simulink subsystem "WindTurbine"  (R2023b)
settings: Solver=VariableStepAuto  StartTime=0.0  StopTime=10.0  RelTol=1e-3
values from neighbouring files (symbols this model uses):
  brakePressure = 100    [wind_turbine_inputs.m]
  generatorEfficiency = 90    [wind_turbine_inputs.m]
  generatorLumpedInductance = 1.9160e-04    (= 0.0001916)    [wind_turbine_inputs.m]
  generatorLumpedResistance = 0.0027    [wind_turbine_inputs.m]
  gridFrequency = 60    [wind_turbine_inputs.m]
  turbineRadius = 70.5/2    (= 35.25)    [wind_turbine_inputs.m]
  turbineRatedPower = 1.5    [wind_turbine_inputs.m]
  wAtGeneratorRatedPower = wTurbineCutOut*gearRatio    (= 1227.93)    [wind_turbine_inputs.m]
undefined symbols (not defined in the file or in its folder): ee_sli_rtmsupport, G, gcbh, X, Y, Z
libraries: sm_lib x42, fl_lib x17, nesl_utility x10, sdl_lib x6, ee_lib x6, simulink x4, eeGeneralControl x3, eeGeneralMeasurement x2
(part 2 of 2)

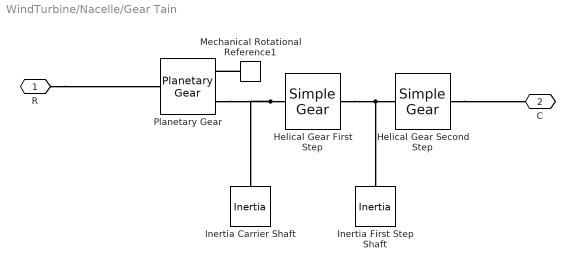
== system WindTurbine/Nacelle/Gear Tain ==
  Helical Gear First Step : sdl_lib/Gears/Simple Gear  ratio=firstStepTeethRatio  rotation_direction=sdl.enum.shaftOutputDirection.opposite  friction_model=sdl.enum.gear_efficiencies_load.constant  T_noload=0.1 N*m  T_nom=5 N*m  efficiency_nom=0.8  efficiency=0.95  temperature_TLU=[ 280 300 320 ] K  load_TLU=[ 1 5 10 ] N*m  efficiency_TLU=[ 0.95 0.9 0.85 ]  efficiency_TLU2=[ 0.85 0.8 0.75; 0.95 0.9 0.85; 0.85 0.8 0.7 ]  w_thr=0.01 rad/s  pwr_thr=0.001 W  enable_backlash=false  hardstop_model=simscape.enum.hardstop.smooth  backlash_distance=1e-3 mm  r_base=0.1 m  transition=1e-4 mm  backlash_stiffness=1e7 N/m  backlash_damping=1e6 N/(m/s)  coeff_rest=0  v_tol=0.001 m/s  f_tol=0 N  mu_visc=[ 0 0 ] N*m/(rad/s)  enable_faults=simscape.enum.onoff.off  efficiency_fault=0.05  external_fault=simscape.enum.onoff.off  temporal_fault=simscape.enum.onoff.off  fault_time=5 s  fault_angles=pi / 12 rad  report_fault=simscape.enum.assert.action.none  thermal_mass=50 J/K  temperature_specify=off  temperature_priority=High  temperature=300 K  temperature_nominal_specify=off  temperature_nominal_unit=K  temperature_nominal_value=1  x_backlash_specify=off  x_backlash_priority=None  x_backlash=0 mm  x_backlash_nominal_specify=off  x_backlash_nominal_unit=mm  x_backlash_nominal_value=1  f_hardstop_specify=off  f_hardstop_priority=None  f_hardstop=0 N  f_hardstop_nominal_specify=off  f_hardstop_nominal_unit=N  f_hardstop_nominal_value=1  v_backlash_specify=off  v_backlash_priority=None  v_backlash=0 m/s  v_backlash_nominal_specify=off  v_backlash_nominal_unit=m/s  v_backlash_nominal_value=1
  Helical Gear Second Step : sdl_lib/Gears/Simple Gear  ratio=secondStepTeethRatio  rotation_direction=sdl.enum.shaftOutputDirection.same  friction_model=sdl.enum.gear_efficiencies_load.constant  T_noload=0.1 N*m  T_nom=5 N*m  efficiency_nom=0.8  efficiency=0.95  temperature_TLU=[ 280 300 320 ] K  load_TLU=[ 1 5 10 ] N*m  efficiency_TLU=[ 0.95 0.9 0.85 ]  efficiency_TLU2=[ 0.85 0.8 0.75; 0.95 0.9 0.85; 0.85 0.8 0.7 ]  w_thr=0.01 rad/s  pwr_thr=0.001 W  enable_backlash=false  hardstop_model=simscape.enum.hardstop.smooth  backlash_distance=1e-3 mm  r_base=0.1 m  transition=1e-4 mm  backlash_stiffness=1e7 N/m  backlash_damping=1e6 N/(m/s)  coeff_rest=0  v_tol=0.001 m/s  f_tol=0 N  mu_visc=[ 0 0 ] N*m/(rad/s)  enable_faults=simscape.enum.onoff.off  efficiency_fault=0.05  external_fault=simscape.enum.onoff.off  temporal_fault=simscape.enum.onoff.off  fault_time=5 s  fault_angles=pi / 12 rad  report_fault=simscape.enum.assert.action.none  thermal_mass=50 J/K  temperature_specify=off  temperature_priority=High  temperature=300 K  temperature_nominal_specify=off  temperature_nominal_unit=K  temperature_nominal_value=1  x_backlash_specify=off  x_backlash_priority=None  x_backlash=0 mm  x_backlash_nominal_specify=off  x_backlash_nominal_unit=mm  x_backlash_nominal_value=1  f_hardstop_specify=off  f_hardstop_priority=None  f_hardstop=0 N  f_hardstop_nominal_specify=off  f_hardstop_nominal_unit=N  f_hardstop_nominal_value=1  v_backlash_specify=off  v_backlash_priority=None  v_backlash=0 m/s  v_backlash_nominal_specify=off  v_backlash_nominal_unit=m/s  v_backlash_nominal_value=1
  Inertia Carrier Shaft : fl_lib/Mechanical/Rotational Elements/Inertia  inertia=carrierShaftInertia kg*m^2  num_ports=foundation.enum.numPorts2.one  w_specify=on  w_priority=None  w=0 rad/s  w_nominal_specify=off  w_nominal_unit=rad/s  w_nominal_value=1  t_specify=off  t_priority=High  t=0 N*m  t_nominal_specify=off  t_nominal_unit=N*m  t_nominal_value=1
  Inertia First Step Shaft : fl_lib/Mechanical/Rotational Elements/Inertia  inertia=stepShaftInertia kg*m^2  num_ports=foundation.enum.numPorts2.one  w_specify=on  w_priority=None  w=0 rad/s  w_nominal_specify=off  w_nominal_unit=rad/s  w_nominal_value=1  t_specify=off  t_priority=High  t=0 N*m  t_nominal_specify=off  t_nominal_unit=N*m  t_nominal_value=1
  Mechanical Rotational Reference1 : fl_lib/Mechanical/Rotational Elements/Mechanical Rotational Reference
  Planetary Gear : sdl_lib/Gears/Planetary Gear  rs_ratio=ringSunTeethRatio  friction_model=sdl.enum.gear_friction.constant  efficiency=[ 0.95 0.95 ]  temperature_TLU=[ 280 300 320 ] K  efficiency_sp_TLU=[ 0.95 0.9 0.85 ]  efficiency_rp_TLU=[ 0.95 0.9 0.85 ]  pwr_thr=[ 0.001 0.001 ] W  mu_visc=[0 0] N*m/(rad/s)  model_inertia=simscape.enum.onoff.off  planet_inertia=0.001 kg*m^2  thermal_mass=50 J/K  T_init=300 K
  R : PMIOPort  Side=Left
  C : PMIOPort  Port=2  Side=Right
  connections:
  Helical Gear First Step/LConn1 -- Inertia First Step Shaft/LConn1 -- Helical Gear Second Step/RConn1
  Mechanical Rotational Reference1/LConn1 -- Planetary Gear/RConn1
  R/RConn1 -- Planetary Gear/LConn1
  Helical Gear First Step/RConn1 -- Inertia Carrier Shaft/LConn1 -- Planetary Gear/RConn2
  Helical Gear Second Step/LConn1 -- C/RConn1

== system WindTurbine/Nacelle/Generator Velocity Sensor  ==
  Ideal Rotational Motion Sensor : fl_lib/Mechanical/Mechanical Sensors/Ideal Rotational Motion Sensor  reference=foundation.enum.MeasurementReference.difference  acceleration_port=false  velocity_port=true  position_port=true  wrap_angle=simscape.enum.onoff.off  offset=0 rad
  Measurement Filter : TransferFcn  Denominator=[0.001 1]
  Mechanical Rotational Reference2 : fl_lib/Mechanical/Rotational Elements/Mechanical Rotational Reference
  PS-Simulink Converter : nesl_utility/PS-Simulink Converter  PhysicalDomain=network_engine_domain  SubClassName=ps_output  LeftPortType=input  RightPortType=output  PseudoPeriodic=off  Frequencies=[]  VectorFormat=1-D array  Unit=rpm  AffineConversion=off
  R : PMIOPort  Side=Left
  wGen : Outport
  wires:
  PS-Simulink Converter/1 -> Measurement Filter/1
  Measurement Filter/1 -> wGen/1
  connections:
  Ideal Rotational Motion Sensor/RConn1 -- Mechanical Rotational Reference2/LConn1
  Ideal Rotational Motion Sensor/LConn1 -- R/RConn1
  Ideal Rotational Motion Sensor/RConn2 -- PS-Simulink Converter/LConn1

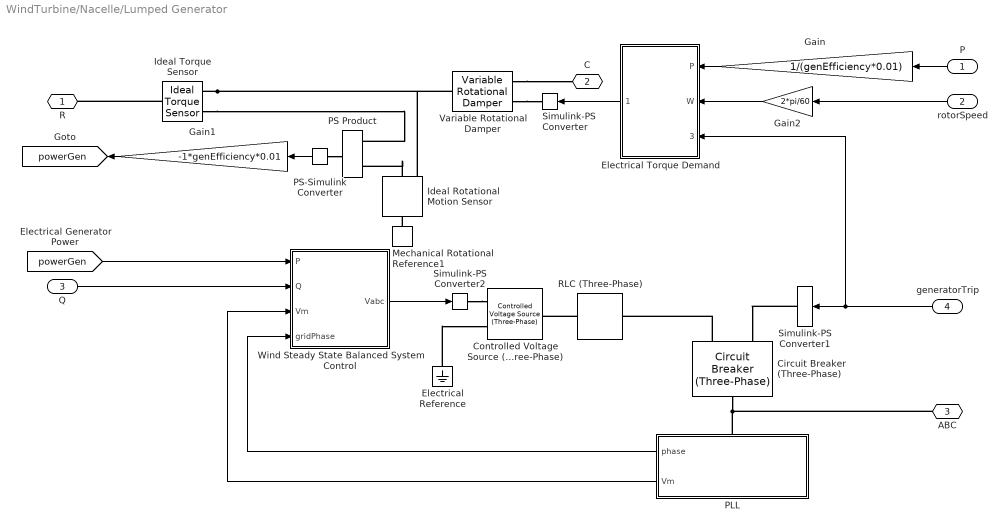
== system WindTurbine/Nacelle/Lumped Generator ==
  P : Inport
  rotorSpeed : Inport  Port=2
  Q : Inport  Port=3
  generatorTrip : Inport  Port=4
  Circuit Breaker (Three-Phase) : ee_lib/Switches & Breakers/Circuit Breaker (Three-Phase)  R_closed=1e-5 Ohm  G_open=1e-8 1/Ohm  threshold=0.5 V  breaker_behavior=ee.enum.switches.breakerBehavior.zeroCrossingEnable
      settings: InternalSimscapePortConfiguration="{\"Bottom\":[],\"Left\":[{\"id\":\"vT\",\"label\":\"vT\",\"type\":\"input\"},{\"id\":\"N1\",\"label\":\"~1\",\"type\":\"foundation.electrical.three_phase\"}],\"Right\":[{\"id\":\"N2\",\"label\":\"~2\",\"type\":\"foundation.electrical.three_phase\"}],\"Top\":[]}"
  Controlled Voltage Source (Three-Phase) : ee_lib/Sources/Controlled Voltage Source (Three-Phase)  input_option=ee.enum.inputType.instantaneous  FRated=60 Hz
      settings: InternalSimscapePortConfiguration="{\"Bottom\":[],\"Left\":[{\"id\":\"S\",\"label\":\"S\",\"type\":\"input\"},{\"id\":\"n\",\"label\":\"n\",\"type\":\"foundation.electrical.electrical\"}],\"Right\":[{\"id\":\"N\",\"label\":\"~\",\"type\":\"foundation.electrical.three_phase\"}],\"Top\":[]}"
  Electrical Reference : fl_lib/Electrical/Electrical Elements/Electrical Reference
  Electrical Torque Demand : Subsystem
  Gain : Gain  Gain=1/(genEfficiency*0.01)
  Gain1 : Gain  Gain=-1*genEfficiency*0.01
  Gain2 : Gain  Gain=2*pi/60
  Ideal Rotational Motion Sensor : fl_lib/Mechanical/Mechanical Sensors/Ideal Rotational Motion Sensor  reference=foundation.enum.MeasurementReference.difference  acceleration_port=false  velocity_port=true  position_port=true  wrap_angle=simscape.enum.onoff.off  offset=0 rad
  Ideal Torque Sensor : fl_lib/Mechanical/Mechanical Sensors/Ideal Torque Sensor
  Mechanical Rotational Reference1 : fl_lib/Mechanical/Rotational Elements/Mechanical Rotational Reference
  PLL : Subsystem
      settings: PortSchema="{\"entries\":[{\"content\":{\"sides\":[{\"content\":{\"connectorIds\":[\"LConn1\"]},\"type\":\"ConnectorPlacement.EquallySpacedRectSide\",\"uuid\":\"d52864e1-db35-4dad-add5-1ee067043f1c\"},{\"content\":{\"connectorIds\":[],\"side\":\"RIGHT\"},\"type\":\"ConnectorPlacement.EquallySpacedRectSide\",\"uuid\":\"a5ba0e67-56ea-44cb-9ec3-4038d29660fe\"},{\"content\":{\"connectorIds\":[],\"side\":\"TOP\"},\"type\":\"ConnectorPlacement.EquallySpacedRectSide\",\"uuid\":\"5a398043-7e81-49e7-beae-eacc9cf31df4\"},{\"content\":{\"connectorIds\":[\"Out1\",\"Out2\"],\"side\":\"BOTTOM\"},\"type\":\"ConnectorPlacement.EquallySpacedRectSide\",\"uuid\":\"36c29948-68bf-4126-b9d0-685ba9cc8aca\"}]},\"type\":\"ConnectorPlacement.EquallySpacedConnector\",\"uuid\":\"348acdbb-59d7-41c8-861d-aa801afd2b04\"}],\"packageUris\":[\"http://schema.mathworks.com/mf0/Connector/R2020b\"],\"version\":\"1.0\"}"
  PS Product : fl_lib/Physical Signals/Functions/PS Product
  PS-Simulink Converter : nesl_utility/PS-Simulink Converter  PhysicalDomain=network_engine_domain  SubClassName=ps_output  LeftPortType=input  RightPortType=output  PseudoPeriodic=off  Frequencies=[]  VectorFormat=inherit  Unit=inherit  AffineConversion=off
  RLC (Three-Phase) : ee_lib/Passive/RLC Assemblies/RLC (Three-Phase)  component_structure=ee.enum.rlc.structure.SeriesRL  R=genResistor Ohm  L=genInductance H  C=1e-6 F  R_parasitic=0 Ohm  G_parasitic=0 1/Ohm  IL_specify=off  IL_priority=High  IL=[0, 0, 0] A  IL_nominal_specify=off  IL_nominal_unit=A  IL_nominal_value=1  VC_specify=off  VC_priority=High  VC=[0, 0, 0] V  VC_nominal_specify=off  VC_nominal_unit=V  VC_nominal_value=1
      settings: InternalSimscapePortConfiguration="{\"Bottom\":[],\"Left\":[{\"id\":\"N1\",\"label\":\"~1\",\"type\":\"foundation.electrical.three_phase\"}],\"Right\":[{\"id\":\"N2\",\"label\":\"~2\",\"type\":\"foundation.electrical.three_phase\"}],\"Top\":[]}"
  Simulink-PS Converter : nesl_utility/Simulink-PS Converter  PhysicalDomain=network_engine_domain  SubClassName=ps_input  LeftPortType=input  RightPortType=output  PseudoPeriodic=off  Frequencies=[]  NoiseDistribution=none  NoiseParameters=[]  Unit=N*m/(rad/s)  AffineConversion=off  FilteringAndDerivatives=provide  SimscapeFilterOrder=1  InputFilterTimeConstant=0.001  UdotUserProvided=0
  Simulink-PS Converter1 : nesl_utility/Simulink-PS Converter  PhysicalDomain=network_engine_domain  SubClassName=ps_input  LeftPortType=input  RightPortType=output  PseudoPeriodic=off  Frequencies=[]  NoiseDistribution=none  NoiseParameters=[]  Unit=V  AffineConversion=off  FilteringAndDerivatives=provide  SimscapeFilterOrder=1  InputFilterTimeConstant=0.001  UdotUserProvided=0
  Simulink-PS Converter2 : nesl_utility/Simulink-PS Converter  PhysicalDomain=network_engine_domain  SubClassName=ps_input  LeftPortType=input  RightPortType=output  PseudoPeriodic=off  Frequencies=[]  NoiseDistribution=none  NoiseParameters=[]  Unit=V  AffineConversion=off  FilteringAndDerivatives=provide  SimscapeFilterOrder=1  InputFilterTimeConstant=0.001  UdotUserProvided=0
  Variable Rotational Damper : sdl_lib/Couplings & Drives/Springs & Dampers/Variable Rotational Damper  Bmin=1e-3 N*m*s/rad
      settings: InternalSimscapePortConfiguration="{\"Bottom\":[],\"Left\":[{\"id\":\"B\",\"label\":\"B\",\"type\":\"input\"},{\"id\":\"R\",\"label\":\"R\",\"type\":\"foundation.mechanical.rotational.rotational\"}],\"Right\":[{\"id\":\"C\",\"label\":\"C\",\"type\":\"foundation.mechanical.rotational.rotational\"}],\"Top\":[]}"
  Wind Steady State Balanced System Control : Subsystem
  R : PMIOPort  Side=Left
  C : PMIOPort  Port=2  Side=Left
  ABC : PMIOPort  Port=3  Side=Right
  tag scope: powerGen=global
  wires:
  generatorTrip/1 -> Electrical Torque Demand/3(generatorTrip), Simulink-PS Converter1/1
  PLL/2(Vm) -> Wind Steady State Balanced System Control/3(Vm)
  [powerGen] -> Wind Steady State Balanced System Control/1(P)
  Gain1/1 -> [powerGen]
  Gain/1 -> Electrical Torque Demand/1(P)
  Gain2/1 -> Electrical Torque Demand/2(W)
  Electrical Torque Demand/1(Damping) -> Simulink-PS Converter/1
  PLL/1(phase) -> Wind Steady State Balanced System Control/4(gridPhase)
  PS-Simulink Converter/1 -> Gain1/1
  rotorSpeed/1 -> Gain2/1
  P/1 -> Gain/1
  Q/1 -> Wind Steady State Balanced System Control/2(Q)
  Wind Steady State Balanced System Control/1(Vabc) -> Simulink-PS Converter2/1
  connections:
  Variable Rotational Damper/LConn2 -- C/RConn1
  Variable Rotational Damper/LConn1 -- Simulink-PS Converter/RConn1
  Simulink-PS Converter1/RConn1 -- Circuit Breaker (Three-Phase)/LConn1
  Circuit Breaker (Three-Phase)/LConn2 -- RLC (Three-Phase)/RConn1
  PLL/LConn1 -- ABC/RConn1 -- Circuit Breaker (Three-Phase)/RConn1
  PS-Simulink Converter/LConn1 -- PS Product/RConn1
  Ideal Rotational Motion Sensor/RConn2 -- PS Product/LConn1
  Electrical Reference/LConn1 -- Controlled Voltage Source (Three-Phase)/LConn2
  Simulink-PS Converter2/RConn1 -- Controlled Voltage Source (Three-Phase)/LConn1
  Mechanical Rotational Reference1/LConn1 -- Ideal Rotational Motion Sensor/LConn1
  Ideal Torque Sensor/RConn2 -- PS Product/LConn2
  Ideal Torque Sensor/LConn1 -- R/RConn1
  Ideal Torque Sensor/RConn1 -- Variable Rotational Damper/RConn1 -- Ideal Rotational Motion Sensor/RConn1
  RLC (Three-Phase)/LConn1 -- Controlled Voltage Source (Three-Phase)/RConn1

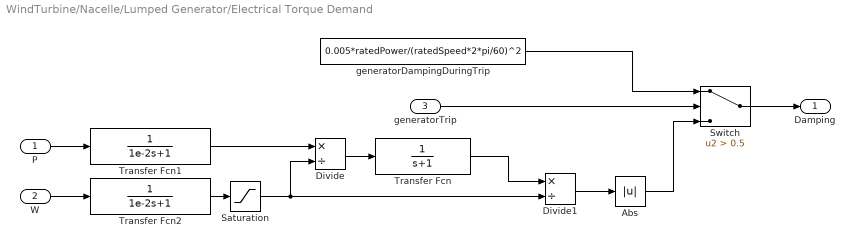
== system WindTurbine/Nacelle/Lumped Generator/Electrical Torque Demand ==
  P : Inport
  W : Inport  Port=2
  generatorTrip : Inport  Port=3
  Abs : Abs  SaturateOnIntegerOverflow=off
  Divide : Product  Inputs=*/
  Divide1 : Product  Inputs=*/
  Saturation : Saturate  UpperLimit=inf  LowerLimit=0.2*ratedSpeed*2*pi/60
  Switch : Switch  Criteria=u2 > Threshold  Threshold=0.5  SaturateOnIntegerOverflow=off  InputSameDT=off
  Transfer Fcn : TransferFcn  Denominator=[1 1]
  Transfer Fcn1 : TransferFcn  Denominator=[1e-2 1]
  Transfer Fcn2 : TransferFcn  Denominator=[1e-2 1]
  generatorDampingDuringTrip : Constant  Value=0.005*ratedPower/(ratedSpeed*2*pi/60)^2
  Damping : Outport
  wires:
  generatorDampingDuringTrip/1 -> Switch/1
  Switch/1 -> Damping/1
  Abs/1 -> Switch/3
  generatorTrip/1 -> Switch/2
  Saturation/1 -> Divide/2, Divide1/2
  Transfer Fcn2/1 -> Saturation/1
  P/1 -> Transfer Fcn1/1
  Transfer Fcn1/1 -> Divide/1
  W/1 -> Transfer Fcn2/1
  Transfer Fcn/1 -> Divide1/1
  Divide/1 -> Transfer Fcn/1
  Divide1/1 -> Abs/1

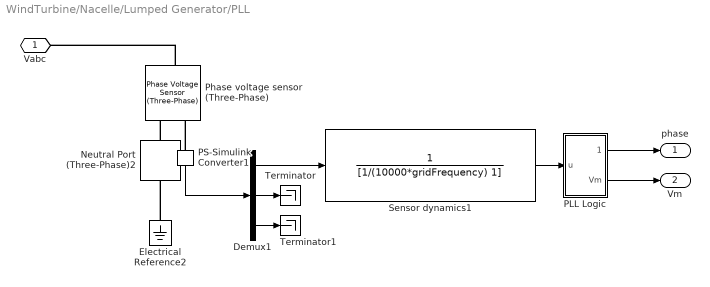
== system WindTurbine/Nacelle/Lumped Generator/PLL ==
  Demux1 : Demux  Outputs=3
  Electrical Reference2 : fl_lib/Electrical/Electrical Elements/Electrical Reference
  Neutral Port (Three-Phase)2 : ee_lib/Connectors & References/Neutral Port (Three-Phase)  G_parasitic=1e-12 1/Ohm
      settings: InternalSimscapePortConfiguration="{\"Bottom\":[],\"Left\":[{\"id\":\"N\",\"label\":\"~\",\"type\":\"foundation.electrical.three_phase\"}],\"Right\":[{\"id\":\"n\",\"label\":\"n\",\"type\":\"foundation.electrical.electrical\"}],\"Top\":[]}"
  PLL Logic : Subsystem
  PS-Simulink Converter1 : nesl_utility/PS-Simulink Converter  PhysicalDomain=network_engine_domain  SubClassName=ps_output  LeftPortType=input  RightPortType=output  PseudoPeriodic=off  Frequencies=[]  VectorFormat=1-D array  Unit=inherit  AffineConversion=off
  Phase voltage sensor (Three-Phase) : ee_lib/Sensors & Transducers/Phase Voltage Sensor (Three-Phase)
  Sensor dynamics1 : TransferFcn  Numerator=1  Denominator=[1/(10000*gridFrequency) 1]
  Terminator : Terminator
  Terminator1 : Terminator
  Vabc : PMIOPort  Side=Left
  phase : Outport
  Vm : Outport  Port=2
  wires:
  PLL Logic/2(Vm) -> Vm/1
  Demux1/2 -> Terminator/1
  Demux1/1 -> Sensor dynamics1/1
  PS-Simulink Converter1/1 -> Demux1/1
  Sensor dynamics1/1 -> PLL Logic/1(u)
  PLL Logic/1(phase) -> phase/1
  Demux1/3 -> Terminator1/1
  connections:
  Phase voltage sensor (Three-Phase)/LConn1 -- Vabc/RConn1
  Electrical Reference2/LConn1 -- Neutral Port (Three-Phase)2/RConn1
  Neutral Port (Three-Phase)2/LConn1 -- Phase voltage sensor (Three-Phase)/RConn2
  PS-Simulink Converter1/LConn1 -- Phase voltage sensor (Three-Phase)/RConn1

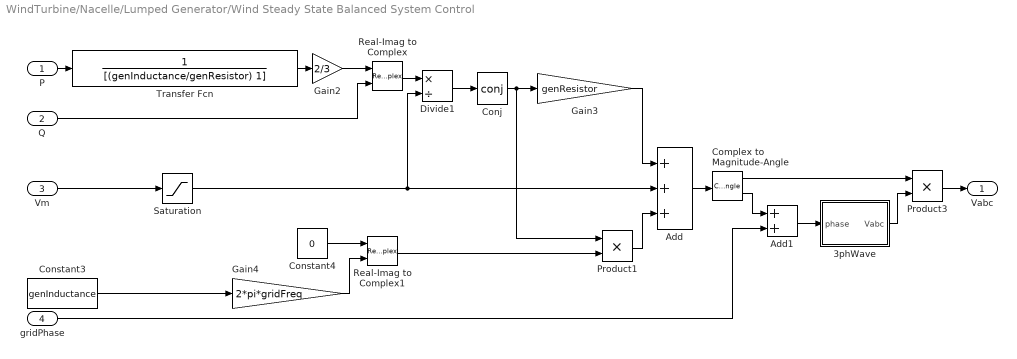
== system WindTurbine/Nacelle/Lumped Generator/Wind Steady State Balanced System Control ==
  P : Inport
  Q : Inport  Port=2
  Vm : Inport  Port=3
  gridPhase : Inport  Port=4
  3phWave : Subsystem
  Add : Sum  Inputs=+++
  Add1 : Sum
  Complex to Magnitude-Angle : ComplexToMagnitudeAngle
  Conj : Math  Operator=conj
  Constant3 : Constant  Value=genInductance
  Constant4 : Constant  Value=0
  Divide1 : Product  Inputs=*/
  Gain2 : Gain  Gain=2/3
  Gain3 : Gain  Gain=genResistor
  Gain4 : Gain  Gain=2*pi*gridFreq
  Product1 : Product
  Product3 : Product
  Real-Imag to Complex : RealImagToComplex
  Real-Imag to Complex1 : RealImagToComplex
  Saturation : Saturate  UpperLimit=10000  LowerLimit=10
  Transfer Fcn : TransferFcn  Denominator=[(genInductance/genResistor) 1]
  Vabc : Outport
  wires:
  P/1 -> Transfer Fcn/1
  Transfer Fcn/1 -> Gain2/1
  Q/1 -> Real-Imag to Complex/2
  Product1/1 -> Add/3
  Vm/1 -> Saturation/1
  Real-Imag to Complex1/1 -> Product1/2
  Constant4/1 -> Real-Imag to Complex1/1
  gridPhase/1 -> Add1/2
  Gain2/1 -> Real-Imag to Complex/1
  Saturation/1 -> Divide1/2, Add/2
  Product3/1 -> Vabc/1
  Conj/1 -> Product1/1, Gain3/1
  Constant3/1 -> Gain4/1
  Real-Imag to Complex/1 -> Divide1/1
  Add/1 -> Complex to Magnitude-Angle/1
  Gain3/1 -> Add/1
  Gain4/1 -> Real-Imag to Complex1/2
  Complex to Magnitude-Angle/1 -> Product3/1
  3phWave/1(Vabc) -> Product3/2
  Complex to Magnitude-Angle/2 -> Add1/1
  Divide1/1 -> Conj/1
  Add1/1 -> 3phWave/1(phase)

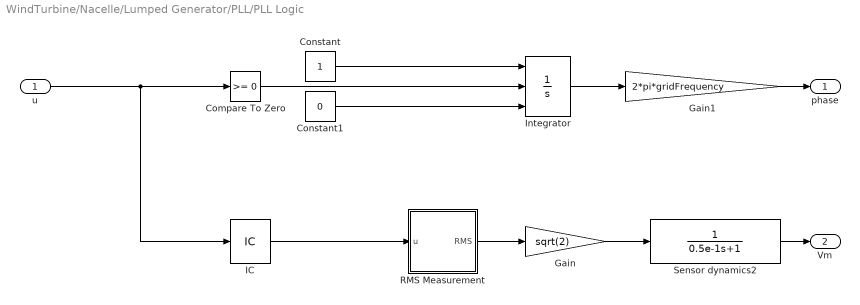
== system WindTurbine/Nacelle/Lumped Generator/PLL/PLL Logic ==
  u : Inport
  Compare To Zero : simulink/Logic and Bit Operations/Compare To Zero  relop=>=  OutDataTypeStr=boolean
  Constant : Constant
  Constant1 : Constant  Value=0
  Gain : Gain  Gain=sqrt(2)
  Gain1 : Gain  Gain=2*pi*gridFrequency
  IC : InitialCondition  Value=1e-4
  Integrator : Integrator  ExternalReset=rising  InitialConditionSource=external  WrapState=on  WrappedStateUpperValue=pi*2  WrappedStateLowerValue=0
  RMS Measurement : Subsystem  LoadFcn=ee_sli_rtmsupport( 'loadfcn', gcbh );  Variant=on  VariantControlMode=label  LabelModeActiveChoice=Total  mask(RMS Measurement){F=gridFrequency, SpecifyHarmonics=off, K=[0 1 2], Ts=0}
      mask prompts: F "physmod:ee:library:comments:control:eeRmsMeasurement:BaseFrequencyHz_MP"; SpecifyHarmonics "physmod:ee:library:comments:control:eeRmsMeasurement:SpecifyHarmonics_MP"; K "physmod:ee:library:comments:control:eeRmsMeasurement:HarmonicNumbers_MP"; Ts "physmod:ee:library:comments:control:eeRmsMeasurement:SampleTime_MP"
      mask help: physmod:ee:library:comments:control:eeRmsMeasurement:RMSMeasurement_MD
      mask init:
      | [timeDomain,G]=ee.mask.initializeRmsMeasurement(gcb,F,Ts,K,SpecifyHarmonics);
      settings: CopyFcn=ee_sli_rtmsupport( 'copyfcn', gcbh );  DeleteFcn=ee_sli_rtmsupport( 'deletefcn', gcbh );  ModelCloseFcn=ee_sli_rtmsupport( 'modelclosefcn', gcbh );  PostSaveFcn=ee_sli_rtmsupport( 'postsavefcn', gcbh );  PreCopyFcn=ee_sli_rtmsupport( 'precopyfcn', gcbh );  OpenFcn=ee_sli_rtmsupport( 'openfcn', gcbh );  CloseFcn=ee_sli_rtmsupport( 'closefcn', gcbh );  PreDeleteFcn=ee_sli_rtmsupport( 'predeletefcn', gcbh );
      mask Help: web(nesl_help(gcbh))
      mask Callback SpecifyHarmonics: ee.mask.callbackRmsMeasurement(gcb);
      mask TypeOptions Ts:
      | Total RMS/Integrator
      | (Discrete or Continuous)/Ts | Total RMS/Periodic Difference
      | (Discrete or Continuous)/Ts | Harmonic RMS/Integrator
      | (Discrete or Continuous)/Ts | Harmonic RMS/SinCos/Integrator with
      | Wrapped State
      | (Discrete or Continuous)/Ts | Harmonic RMS/Periodic Difference
      | (Discrete or Continuous)/Ts
      mask DialogControl F Prompt: Base frequency (Hz)
      mask DialogControl SpecifyHarmonics Prompt: Specify harmonics
      mask DialogControl K Prompt: Harmonic numbers
      mask DialogControl Ts Prompt: Sample time
      mask Display: ee.mask.drawRmsMeasurement;
  Sensor dynamics2 : TransferFcn  Numerator=1  Denominator=[0.5e-1 1]
  phase : Outport
  Vm : Outport  Port=2
  wires:
  u/1 -> Compare To Zero/1, IC/1
  Sensor dynamics2/1 -> Vm/1
  IC/1 -> RMS Measurement/1(u)
  Gain/1 -> Sensor dynamics2/1
  RMS Measurement/1(RMS) -> Gain/1
  Gain1/1 -> phase/1
  Constant1/1 -> Integrator/3
  Compare To Zero/1 -> Integrator/2
  Constant/1 -> Integrator/1
  Integrator/1 -> Gain1/1

== system WindTurbine/Nacelle/Lumped Generator/Wind Steady State Balanced System Control/3phWave ==
  phase : Inport
  Add Constant : Bias  Bias=-120*pi/180  SaturateOnIntegerOverflow=off
  Add Constant1 : Bias  Bias=120*pi/180  SaturateOnIntegerOverflow=off
  Mux : Mux  Inputs=3
  Trigonometric Function : Trigonometry
  Vabc : Outport
  wires:
  Trigonometric Function/1 -> Vabc/1
  Add Constant1/1 -> Mux/3
  Add Constant/1 -> Mux/2
  phase/1 -> Mux/1, Add Constant/1, Add Constant1/1
  Mux/1 -> Trigonometric Function/1

== system WindTurbine/Nacelle/Lumped Generator/PLL/PLL Logic/RMS Measurement ==
  u : Inport
  Harmonic RMS : Subsystem  VariantControl=Harmonic
  Total RMS : Subsystem  VariantControl=Total
  RMS : Outport  VectorParamsAs1DForOutWhenUnconnected=off

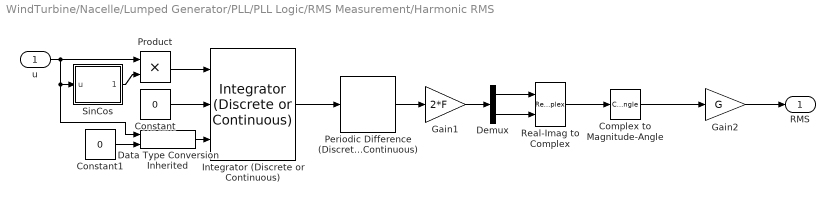
== system WindTurbine/Nacelle/Lumped Generator/PLL/PLL Logic/RMS Measurement/Harmonic RMS ==
  u : Inport
  Complex to Magnitude-Angle : ComplexToMagnitudeAngle  Output=Magnitude
  Constant : Constant  Value=0
  Constant1 : Constant  Value=0
  Data Type Conversion Inherited : simulink/Signal Attributes/Data Type Conversion Inherited  ConvertRealWorld=Real World Value  DoSatur=off
  Demux : Demux  Outputs=2
  Gain1 : Gain  Gain=2*F
  Gain2 : Gain  Gain=G
  Integrator (Discrete or Continuous) : eeGeneralControl/Integrator (Discrete or Continuous)  LabelModeActiveChoice=Continuous  ExternalReset=level  LimitType=Anti-windup  B=inf  A=-inf  Ts=Ts
  Periodic Difference (Discrete or Continuous) : eeGeneralMeasurement/Periodic Difference (Discrete or Continuous)  LabelModeActiveChoice=Continuous  F=F  Ts=Ts
  Product : Product
  Real-Imag to Complex : RealImagToComplex
  SinCos : Subsystem
  RMS : Outport  VectorParamsAs1DForOutWhenUnconnected=off
  wires:
  Complex to Magnitude-Angle/1 -> Gain2/1
  Product/1 -> Integrator (Discrete or Continuous)/1
  Gain1/1 -> Demux/1
  SinCos/1(SinCos) -> Product/2
  Demux/1 -> Real-Imag to Complex/1
  Real-Imag to Complex/1 -> Complex to Magnitude-Angle/1
  Periodic Difference (Discrete or Continuous)/1 -> Gain1/1
  u/1 -> Product/1, Data Type Conversion Inherited/1, SinCos/1(u)
  Demux/2 -> Real-Imag to Complex/2
  Gain2/1 -> RMS/1
  Constant/1 -> Integrator (Discrete or Continuous)/2
  Integrator (Discrete or Continuous)/1 -> Periodic Difference (Discrete or Continuous)/1
  Data Type Conversion Inherited/1 -> Integrator (Discrete or Continuous)/3
  Constant1/1 -> Data Type Conversion Inherited/2

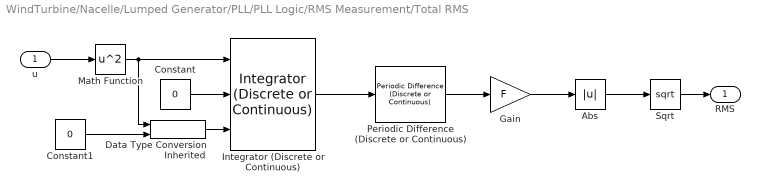
== system WindTurbine/Nacelle/Lumped Generator/PLL/PLL Logic/RMS Measurement/Total RMS ==
  u : Inport
  Abs : Abs  SaturateOnIntegerOverflow=off
  Constant : Constant  Value=0
  Constant1 : Constant  Value=0
  Data Type Conversion Inherited : simulink/Signal Attributes/Data Type Conversion Inherited  ConvertRealWorld=Real World Value  DoSatur=off
  Gain : Gain  Gain=F
  Integrator (Discrete or Continuous) : eeGeneralControl/Integrator (Discrete or Continuous)  LabelModeActiveChoice=Continuous  ExternalReset=level  LimitType=Anti-windup  B=inf  A=-inf  Ts=Ts
  Math Function : Math  Operator=square  SignedPower=on
  Periodic Difference (Discrete or Continuous) : eeGeneralMeasurement/Periodic Difference (Discrete or Continuous)  LabelModeActiveChoice=Continuous  F=F  Ts=Ts
  Sqrt : Sqrt
  RMS : Outport  VectorParamsAs1DForOutWhenUnconnected=off
  wires:
  Abs/1 -> Sqrt/1
  Gain/1 -> Abs/1
  Constant/1 -> Integrator (Discrete or Continuous)/2
  Math Function/1 -> Data Type Conversion Inherited/1, Integrator (Discrete or Continuous)/1
  u/1 -> Math Function/1
  Integrator (Discrete or Continuous)/1 -> Periodic Difference (Discrete or Continuous)/1
  Sqrt/1 -> RMS/1
  Periodic Difference (Discrete or Continuous)/1 -> Gain/1
  Data Type Conversion Inherited/1 -> Integrator (Discrete or Continuous)/3
  Constant1/1 -> Data Type Conversion Inherited/2

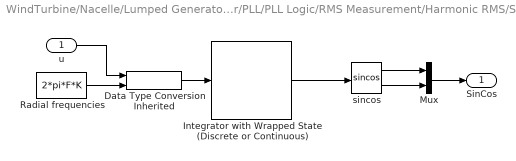
== system WindTurbine/Nacelle/Lumped Generator/PLL/PLL Logic/RMS Measurement/Harmonic RMS/SinCos ==
  u : Inport
  Data Type Conversion Inherited : simulink/Signal Attributes/Data Type Conversion Inherited  ConvertRealWorld=Real World Value  DoSatur=off
  Integrator with Wrapped State (Discrete or Continuous) : eeGeneralControl/Integrator with Wrapped State (Discrete or Continuous)  LabelModeActiveChoice=Continuous  WrappedStateUpperValue=2*pi  WrappedStateLowerValue=0  x0=0  Ts=Ts
  Mux : Mux  Inputs=2
  Radial frequencies : Constant  Value=2*pi*F*K
  sincos : Trigonometry  Operator=sincos
  SinCos : Outport  VectorParamsAs1DForOutWhenUnconnected=off
  wires:
  sincos/2 -> Mux/2
  sincos/1 -> Mux/1
  Mux/1 -> SinCos/1
  Integrator with Wrapped State (Discrete or Continuous)/1 -> sincos/1
  Data Type Conversion Inherited/1 -> Integrator with Wrapped State (Discrete or Continuous)/1
  Radial frequencies/1 -> Data Type Conversion Inherited/2
  u/1 -> Data Type Conversion Inherited/1
